simulink model "Masina_distanta"  (Simulink 7.6)
settings: Solver=ode3  StartTime=0.0  StopTime=300  FixedStep=1  RelTol=1e-3
libraries: simulink_need_slupdate x1, simulink x1
settings Model: Creator=Bogdy  LastModifiedBy=Bogdy
settings OptimizationCC: InlineInvariantSignals=on  InitFltsAndDblsToZero=on
settings DebuggingCC: SaveWithParameterizedLinksMsg=none  SignalResolutionControl=TryResolveAllWithWarning  MultiTaskDSMMsg=warning  MultiTaskCondExecSysMsg=none  StrictBusMsg=None
settings RTWCC: IncludeERTFirstTime=on
settings GRTTargetCC: TargetFcnLib=ansi_tfl_tmw.mat

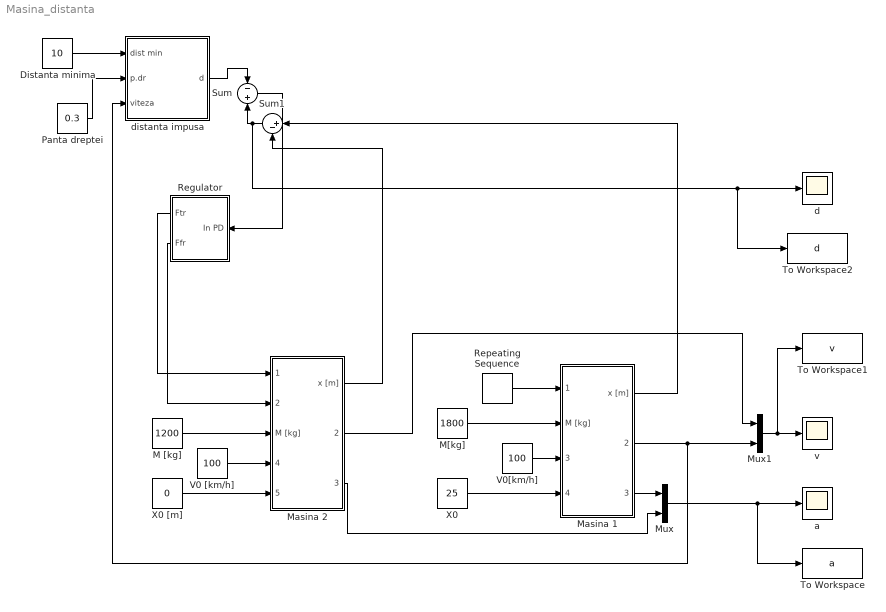
== system Masina_distanta ==
  Distanta minima : Constant  Value=10
  M [kg] : Constant  Value=1200
  M[kg] : Constant  Value=1800
  Masina 1 : Subsystem
  Masina 2 : Subsystem
  Mux : Mux  Inputs=2
  Mux1 : Mux  Inputs=2
  Panta dreptei : Constant  Value=0.3
  Regulator : Subsystem
  Repeating Sequence : simulink/Sources/Repeating Sequence  SystemSampleTime=-1  rep_seq_t=[0 1 5 10 20 30 40 50 59 60]  rep_seq_y=[1 4 4 0 -2 -3 1 2 -1 1]
  Sum : Sum  Inputs=-+
  Sum1 : Sum  Inputs=|+-
  To Workspace : ToWorkspace  VariableName=a  SampleTime=-1  SaveFormat=Array
  To Workspace1 : ToWorkspace  VariableName=v  SampleTime=-1  SaveFormat=Array
  To Workspace2 : ToWorkspace  VariableName=d  SampleTime=-1  SaveFormat=Array
  V0 [km/h] : Constant  Value=100
  V0[km/h] : Constant  Value=100
  X0 : Constant  Value=25
  X0 [m] : Constant  Value=0
  a : Scope
      settings: TimeRange=60  YMin=0  YMax=550
  d : Scope
      settings: TimeRange=60  YMin=0  YMax=550  SaveName=ScopeData2
  distanta impusa : Subsystem
  v : Scope
      settings: TimeRange=19.19999999999999  YMin=181.375  YMax=182.375  SaveName=ScopeData3
  wires:
  Panta dreptei/1 -> distanta impusa/2(p.dr)
  V0 [km/h]/1 -> Masina 2/4(V0 [km/h])
  X0 [m]/1 -> Masina 2/5(X0 [m])
  Sum1/1 -> Sum/2, d/1, To Workspace2/1
  Mux/1 -> a/1, To Workspace/1
  Mux1/1 -> v/1, To Workspace1/1
  Distanta minima/1 -> distanta impusa/1(dist min)
  distanta impusa/1(d) -> Sum/1
  M [kg]/1 -> Masina 2/3(M [kg])
  Sum/1 -> Regulator/1(In PD)
  Repeating Sequence/1 -> Masina 1/1(Ftr [kN])
  M[kg]/1 -> Masina 1/2(M [kg])
  V0[km/h]/1 -> Masina 1/3(V0 [km/h])
  X0/1 -> Masina 1/4(X0 [m])
  Masina 1/1(x [m]) -> Sum1/1
  Masina 2/1(x [m]) -> Sum1/2
  Regulator/1(Ftr) -> Masina 2/1(Ftr [kN])
  Regulator/2(Ffr) -> Masina 2/2(Ffr [kN])
  Masina 1/2(v [km/h]) -> distanta impusa/3(viteza), Mux1/2
  Masina 1/3(a [m/s2]) -> Mux/1
  Masina 2/3(a [m/s2]) -> Mux/2
  Masina 2/2(v [km/h]) -> Mux1/1

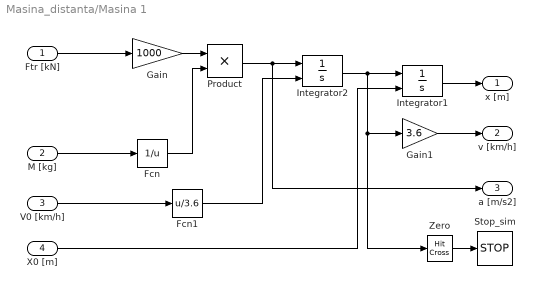
== system Masina_distanta/Masina 1 ==
  Ftr [kN] : Inport
  M [kg] : Inport  Port=2
  V0 [km/h] : Inport  Port=3
  X0 [m] : Inport  Port=4
  Fcn : Fcn  Expr=1/u
  Fcn1 : Fcn  Expr=u/3.6
  Gain : Gain  Gain=1000  SaturateOnIntegerOverflow=on  OutDataTypeStr=Inherit: Same as input  ParamDataTypeStr=Inherit: Same as input
  Gain1 : Gain  Gain=3.6  SaturateOnIntegerOverflow=on  OutDataTypeStr=Inherit: Same as input  ParamDataTypeStr=Inherit: Same as input
  Integrator1 : Integrator  InitialConditionSource=external
  Integrator2 : Integrator  InitialConditionSource=external
  Product : Product  SaturateOnIntegerOverflow=on  RndMeth=Zero  InputSameDT=on  OutDataTypeStr=Inherit: Same as first input
  Stop_sim : Stop
  Zero : HitCross  HitCrossingOffset=1  HitCrossingDirection=falling
  x [m] : Outport
  v [km/h] : Outport  Port=2
  a [m/s2] : Outport  Port=3
  wires:
  M [kg]/1 -> Fcn/1
  Fcn/1 -> Product/2
  Product/1 -> a [m/s2]/1, Integrator2/1
  V0 [km/h]/1 -> Fcn1/1
  Integrator2/1 -> Integrator1/1, Gain1/1, Zero/1
  X0 [m]/1 -> Integrator1/2
  Integrator1/1 -> x [m]/1
  Fcn1/1 -> Integrator2/2
  Gain1/1 -> v [km/h]/1
  Zero/1 -> Stop_sim/1
  Ftr [kN]/1 -> Gain/1
  Gain/1 -> Product/1

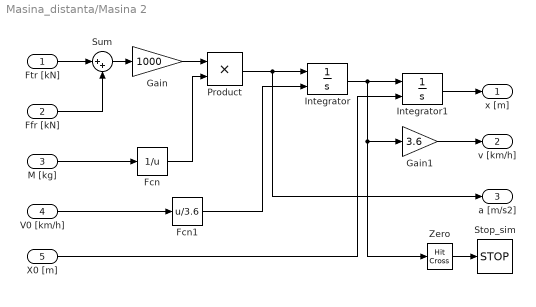
== system Masina_distanta/Masina 2 ==
  Ftr [kN] : Inport
  Ffr [kN] : Inport  Port=2
  M [kg] : Inport  Port=3
  V0 [km/h] : Inport  Port=4
  X0 [m] : Inport  Port=5
  Fcn : Fcn  Expr=1/u
  Fcn1 : Fcn  Expr=u/3.6
  Gain : Gain  Gain=1000  SaturateOnIntegerOverflow=on  OutDataTypeStr=Inherit: Same as input  ParamDataTypeStr=Inherit: Same as input
  Gain1 : Gain  Gain=3.6  SaturateOnIntegerOverflow=on  OutDataTypeStr=Inherit: Same as input  ParamDataTypeStr=Inherit: Same as input
  Integrator : Integrator  InitialConditionSource=external
  Integrator1 : Integrator  InitialConditionSource=external
  Product : Product  SaturateOnIntegerOverflow=on  RndMeth=Zero  InputSameDT=on  OutDataTypeStr=Inherit: Same as first input
  Stop_sim : Stop
  Sum : Sum  Inputs=|++  SaturateOnIntegerOverflow=on  InputSameDT=on  OutDataTypeStr=Inherit: Same as first input
  Zero : HitCross  HitCrossingOffset=1  HitCrossingDirection=falling
  x [m] : Outport
  v [km/h] : Outport  Port=2
  a [m/s2] : Outport  Port=3
  wires:
  Ffr [kN]/1 -> Sum/2
  M [kg]/1 -> Fcn/1
  Sum/1 -> Gain/1
  Fcn/1 -> Product/2
  Product/1 -> Integrator/1, a [m/s2]/1
  V0 [km/h]/1 -> Fcn1/1
  Integrator/1 -> Integrator1/1, Gain1/1, Zero/1
  X0 [m]/1 -> Integrator1/2
  Integrator1/1 -> x [m]/1
  Fcn1/1 -> Integrator/2
  Gain1/1 -> v [km/h]/1
  Zero/1 -> Stop_sim/1
  Ftr [kN]/1 -> Sum/1
  Gain/1 -> Product/1

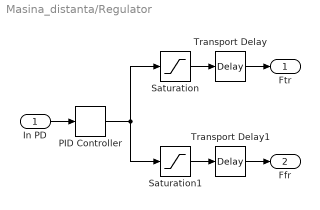
== system Masina_distanta/Regulator ==
  In PD : Inport
  PID Controller : simulink_need_slupdate/PID Controller  SystemSampleTime=-1  P=15  I=0  D=70
  Saturation : Saturate  UpperLimit=4  LowerLimit=0
  Saturation1 : Saturate  UpperLimit=0  LowerLimit=-4
  Transport Delay : TransportDelay  DelayTime=0.1
  Transport Delay1 : TransportDelay  DelayTime=0.1
  Ftr : Outport
  Ffr : Outport  Port=2
  wires:
  Saturation1/1 -> Transport Delay1/1
  Saturation/1 -> Transport Delay/1
  PID Controller/1 -> Saturation/1, Saturation1/1
  Transport Delay/1 -> Ftr/1
  In PD/1 -> PID Controller/1
  Transport Delay1/1 -> Ffr/1

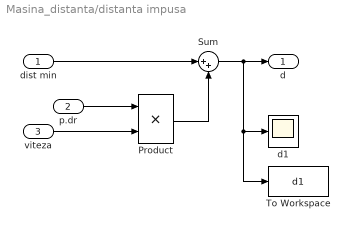
== system Masina_distanta/distanta impusa ==
  dist min : Inport
  p.dr : Inport  Port=2
  viteza : Inport  Port=3
  Product : Product  RndMeth=Zero
  Sum : Sum  Inputs=|++
  To Workspace : ToWorkspace  VariableName=d1  SampleTime=-1  SaveFormat=Array
  d1 : Scope
      settings: TimeRange=60  YMin=0  YMax=550
  d : Outport
  wires:
  dist min/1 -> Sum/1
  Product/1 -> Sum/2
  p.dr/1 -> Product/1
  Sum/1 -> d/1, d1/1, To Workspace/1
  viteza/1 -> Product/2
